simulink model "model"  (R2025b)
settings: Solver=FixedStepAuto  StartTime=0.0  StopTime=20  FixedStep=0.01  RelTol=1e-3
model workspace (MAT data in the model file):
  freq = 0.87
values from neighbouring files (symbols this model uses):
  pwm = k * 125    [measureMotorDiff.m]    (also in modelSetup.m = 2000)
settings Model: Creator=marko  LastModifiedBy=marko
settings DebuggingCC: UnconnectedInputMsg=warning  UnconnectedOutputMsg=warning  UnconnectedLineMsg=warning
settings ModelReferenceCC: EnableRefExpFcnMdlSchedulingChecks=on
settings RTWCC: GPUComputeCapability=3.5  DLArmComputeVersion=19.05

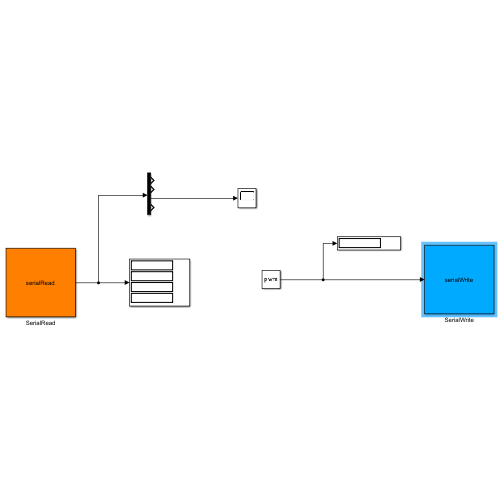
[thumbnail: Simulink's stored preview of the top-level diagram]
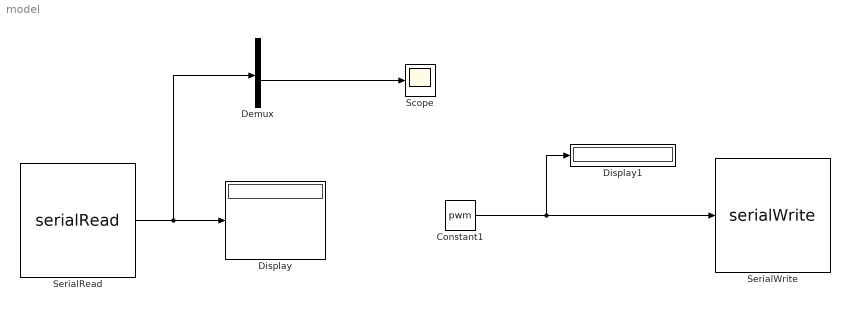
== system model ==
  Constant1 : Constant  Value=pwm
  Demux : Demux
  Display : Display
  Display1 : Display
  Scope : Scope
      settings: TimeSpan=500  ActiveDisplayYMinimum=-10.10013  ActiveDisplayYMaximum=78.16413
  SerialRead : M-S-Function  FunctionName=serialRead  Parameters='COM3'
  SerialWrite : M-S-Function  FunctionName=serialWrite  Parameters='COM3'
  wires:
  SerialRead/1 -> Demux/1, Display/1
  Constant1/1 -> SerialWrite/1, Display1/1
  Demux/3 -> Scope/1
